simulink model "lab4_2018b"  (R2018b)
settings: Solver=VariableStepAuto  StartTime=0.0  StopTime=150  MaxStep=1e-3  RelTol=1e-3
undefined symbols (not defined in the file): a, b, c, d
settings Model: Creator=Bernard  LastModifiedBy=wangh
settings DataIOCC: ReturnWorkspaceOutputs=on

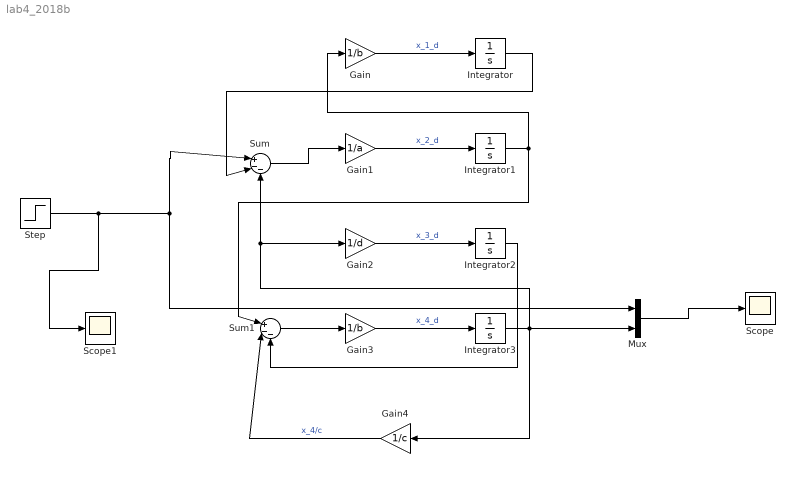
== system lab4_2018b ==
  Gain : Gain  Gain=1/b
  Gain1 : Gain  Gain=1/a
  Gain2 : Gain  Gain=1/d
  Gain3 : Gain  Gain=1/b
  Gain4 : Gain  Gain=1/c
  Integrator{,1..3} (4 alike) : Integrator
  Mux : Mux  Inputs=2
  Scope : Scope
  Scope1 : Scope
  Step : Step  SampleTime=0
  Sum : Sum  Inputs=|+--
  Sum1 : Sum  Inputs=|+--
  wires:
  Gain/1 -> Integrator/1  "x_1_d"
  Integrator1/1 -> Sum1/1, Gain/1
  Gain1/1 -> Integrator1/1  "x_2_d"
  Step/1 -> Scope1/1, Mux/1, Sum/1
  Integrator/1 -> Sum/2
  Sum/1 -> Gain1/1
  Integrator3/1 -> Mux/2, Gain4/1, Gain2/1, Sum/3
  Gain2/1 -> Integrator2/1  "x_3_d"
  Gain3/1 -> Integrator3/1  "x_4_d"
  Sum1/1 -> Gain3/1
  Integrator2/1 -> Sum1/3
  Gain4/1 -> Sum1/2  "x_4/c"
  Mux/1 -> Scope/1
